simulink model "EB_12B"  (R2021b)
settings: Solver=ode3  StartTime=0.0  StopTime=0  FixedStep=.01  RelTol=1e-3  EnableMultiTasking=on
model workspace (MAT data in the model file):
  I = [1  0  0; 0  1  0; 0  0  1]
  I0 = [0  0  0; 0  0  0; 0  0  0]
  N = 18
  Wp = [1  0  0  0  0; 0  1  0  0  0; 0  0  1  0  0; 0  0  0  1  0; 0  0  0  0  1]
  X = [-0.000916135593528 0.000741784354662 -0.000111198836647 -0.000114918934981 -0.000338802758293 0.00087934621238 0.000425682524619 0.000877814042518 6.19118807071e-05 -0.000956394036441 0.000640782162368 -0.000425007884451 0.000734759332255 0.000720421624474 0.000101264737043]
  cmd.Wp = [1  0  0  0  0; 0  1  0  0  0; 0  0  1  0  0; 0  0  0  1  0; 0  0  0  0  1]
  cmd.d = [3; -1; 2]
  cmd.up = [0; 0; 0; 0; 0]
  cmd.I0 = [0  0  0; 0  0  0; 0  0  0]
  cmd.I = [1  0  0; 0  1  0; 0  0  1]
  cmd.tout = 0
  cs : handle (value not decoded)
  curPath = '/Users/khouloud.gaaloul/Documents/Projects/QRA-LocalSearch/Local Search Algorithms/Problems'
  d = 16
  hws = [3707764736; 2; 1; 1; 1; 1]
  i = 7
  j = 5
  list(1).name = 'I'
  list(1).size = [3 3]
  list(1).bytes = 72
  list(1).class = 'double'
  list(1).global = 0
  list(1).sparse = 0
  list(1).complex = 0
  list(1).nesting.function = ''
  list(1).nesting.level = 1
  list(1).persistent = 0
  list(2).name = 'I0'
  list(2).size = [3 3]
  list(2).bytes = 72
  list(2).class = 'double'
  list(2).global = 0
  list(2).sparse = 0
  list(2).complex = 0
  list(2).nesting.function = ''
  list(2).nesting.level = 1
  list(2).persistent = 0
  list(3).name = 'N'
  list(3).size = [1 1]
  list(3).bytes = 8
  list(3).class = 'double'
  list(3).global = 0
  list(3).sparse = 0
  list(3).complex = 0
  list(3).nesting.function = ''
  list(3).nesting.level = 1
  list(3).persistent = 0
  list(4).name = 'Wp'
  list(4).size = [5 5]
  list(4).bytes = 200
  list(4).class = 'double'
  list(4).global = 0
  list(4).sparse = 0
  list(4).complex = 0
  list(4).nesting.function = ''
  list(4).nesting.level = 1
  list(4).persistent = 0
  list(5).name = 'cs'
  list(5).size = [1 1]
  list(5).bytes = 0
  list(5).class = 'Simulink.ConfigSet'
  list(5).global = 0
  list(5).sparse = 0
  list(5).complex = 0
  list(5).nesting.function = ''
  list(5).nesting.level = 1
  list(5).persistent = 0
  list(6).name = 'curPath'
  list(6).size = [1 91]
  list(6).bytes = 182
  list(6).class = 'char'
  list(6).global = 0
  list(6).sparse = 0
  list(6).complex = 0
  list(6).nesting.function = ''
  list(6).nesting.level = 1
  list(6).persistent = 0
  list(7).name = 'd'
  list(7).size = [3 1]
  list(7).bytes = 24
  list(7).class = 'double'
  list(7).global = 0
  list(7).sparse = 0
  list(7).complex = 0
  list(7).nesting.function = ''
  list(7).nesting.level = 1
  list(7).persistent = 0
  list(8).name = 'hws'
  list(8).size = [1 1]
  list(8).bytes = 8
  list(8).class = 'Simulink.ModelWorkspace'
  list(8).global = 0
  list(8).sparse = 0
  list(8).complex = 0
  list(8).nesting.function = ''
  list(8).nesting.level = 1
  list(8).persistent = 0
  list(9).name = 'i'
  list(9).size = [1 1]
  list(9).bytes = 8
  list(9).class = 'double'
  list(9).global = 0
  list(9).sparse = 0
  list(9).complex = 0
  list(9).nesting.function = ''
  list(9).nesting.level = 1
  list(9).persistent = 0
  list(10).name = 'j'
  list(10).size = [1 1]
  list(10).bytes = 8
  list(10).class = 'double'
  list(10).global = 0
  list(10).sparse = 0
  list(10).complex = 0
  list(10).nesting.function = ''
  list(10).nesting.level = 1
  list(10).persistent = 0
  list(11).name = 'list'
  list(11).size = [18 1]
  list(11).bytes = 26158
  list(11).class = 'struct'
  list(11).global = 0
  list(11).sparse = 0
  list(11).complex = 0
  list(11).nesting.function = ''
  list(11).nesting.level = 1
  list(11).persistent = 0
  list(12).name = 'model_cs'
  list(12).size = [1 1]
  list(12).bytes = 0
  list(12).class = 'Simulink.ConfigSet'
  list(12).global = 0
  list(12).sparse = 0
  list(12).complex = 0
  list(12).nesting.function = ''
  list(12).nesting.level = 1
  list(12).persistent = 0
  list(13).name = 'modelpath'
  list(13).size = [1 80]
  list(13).bytes = 160
  list(13).class = 'char'
  list(13).global = 0
  list(13).sparse = 0
  list(13).complex = 0
  list(13).nesting.function = ''
  list(13).nesting.level = 1
  list(13).persistent = 0
  list(14).name = 'simOut'
  list(14).size = [1 1]
  list(14).bytes = 10925
  list(14).class = 'Simulink.SimulationOutput'
  list(14).global = 0
  list(14).sparse = 0
  list(14).complex = 0
  list(14).nesting.function = ''
  list(14).nesting.level = 1
  list(14).persistent = 0
  list(15).name = 'tout'
  list(15).size = [1 1]
  list(15).bytes = 8
  list(15).class = 'double'
  list(15).global = 0
  list(15).sparse = 0
  list(15).complex = 0
  list(15).nesting.function = ''
  list(15).nesting.level = 1
  list(15).persistent = 0
  list(16).name = 'up'
  list(16).size = [5 1]
  list(16).bytes = 40
  list(16).class = 'double'
  list(16).global = 0
  list(16).sparse = 0
  list(16).complex = 0
  list(16).nesting.function = ''
  list(16).nesting.level = 1
  list(16).persistent = 0
  list(17).name = 'var'
  list(17).size = [3 5]
  list(17).bytes = 120
  list(17).class = 'double'
  list(17).global = 0
  list(17).sparse = 0
  list(17).complex = 0
  list(17).nesting.function = ''
  list(17).nesting.level = 1
  list(17).persistent = 0
  list(18).name = 'varout'
  list(18).size = [1 1]
  list(18).bytes = 4323
  list(18).class = 'struct'
  list(18).global = 0
  list(18).sparse = 0
  list(18).complex = 0
  list(18).nesting.function = ''
  list(18).nesting.level = 1
  list(18).persistent = 0
  model_cs : handle (value not decoded)
  modelpath = '/Users/khouloud.gaaloul/Documents/Projects/QRA-LocalSearch/Simulink Models/6_eb/'
  req = 'R2'
  simOut = Simulink.SimulationOutput
  simOut.Data.tout = 0
  simOut.Data.varout.time = 0
  simOut.Data.varout.signals(1).values = [0  0  0; 0  0  0; 0  0  0]
  simOut.Data.varout.signals(1).dimensions = [3 3]
  simOut.Data.varout.signals(1).label = ''
  simOut.Data.varout.signals(1).blockName = 'EB_12B/check'
  simOut.Data.varout.signals(2).values = [1000000000000  0  0; 0  1000000000000  0; 0  0  1000000000000]
  simOut.Data.varout.signals(2).dimensions = [3 3]
  simOut.Data.varout.signals(2).label = ''
  simOut.Data.varout.signals(2).blockName = 'EB_12B/yinv'
  simOut.Data.varout.signals(3).values = [0  0  0; 0  0  0; 0  0  0; 0  0  0; 0  0  0]
  simOut.Data.varout.signals(3).dimensions = [5 3]
  simOut.Data.varout.signals(3).label = ''
  simOut.Data.varout.signals(3).blockName = 'EB_12B/P'
  simOut.Data.varout.signals(4).values = [0 0 0 0 0]
  simOut.Data.varout.signals(4).dimensions = 5
  simOut.Data.varout.signals(4).label = ''
  simOut.Data.varout.signals(4).blockName = 'EB_12B/u'
  simOut.Data.varout.signals(5).values = [-3 1 -2]
  simOut.Data.varout.signals(5).dimensions = 3
  simOut.Data.varout.signals(5).label = ''
  simOut.Data.varout.signals(5).blockName = 'EB_12B/Buminusd'
  simOut.Data.varout.signals(6).values = 0
  simOut.Data.varout.signals(6).dimensions = 1
  simOut.Data.varout.signals(6).label = ''
  simOut.Data.varout.signals(6).blockName = 'EB_12B/J'
  simOut.Data.varout.signals(7).values = 1
  simOut.Data.varout.signals(7).dimensions = 1
  simOut.Data.varout.signals(7).label = ''
  simOut.Data.varout.signals(7).blockName = 'EB_12B/ridge_on'
  simOut.Metadata = Simulink.SimulationMetadata
  simOut.Metadata.ModelInfo.ModelName = 'EB_12B'
  simOut.Metadata.ModelInfo.ModelVersion = '1.70'
  simOut.Metadata.ModelInfo.ModelFilePath = '/Users/khouloud.gaaloul/Documents/Projects/QRA-LocalSearch/Simulink Models/6_eb/EB_12B.slx'
  simOut.Metadata.ModelInfo.UserID = 'khouloud.gaaloul'
  simOut.Metadata.ModelInfo.MachineName = ''
  simOut.Metadata.ModelInfo.Platform = 'MACI64'
  simOut.Metadata.ModelInfo.ModelStructuralChecksum = [893138603; 2259620877; 265752267; 1923685794]
  simOut.Metadata.ModelInfo.SimulationMode = 'normal'
  simOut.Metadata.ModelInfo.StartTime = 0
  simOut.Metadata.ModelInfo.StopTime = 0
  simOut.Metadata.ModelInfo.SolverInfo.Type = 'Fixed-Step'
  simOut.Metadata.ModelInfo.SolverInfo.Solver = 'FixedStepDiscrete'
  simOut.Metadata.ModelInfo.SolverInfo.FixedStepSize = 0.01
  simOut.Metadata.ModelInfo.SimulinkVersion.Name = 'Simulink'
  simOut.Metadata.ModelInfo.SimulinkVersion.Version = '9.1'
  simOut.Metadata.ModelInfo.SimulinkVersion.Release = '(R2018a)'
  simOut.Metadata.ModelInfo.SimulinkVersion.Date = '06-Feb-2018'
  simOut.Metadata.ModelInfo.LoggingInfo.LoggingToFile = 'off'
  simOut.Metadata.TimingInfo.WallClockTimestampStart = '2018-11-07 17:57:54.082518'
  simOut.Metadata.TimingInfo.WallClockTimestampStop = '2018-11-07 17:57:54.533264'
  simOut.Metadata.TimingInfo.InitializationElapsedWallTime = 0.383556
  simOut.Metadata.TimingInfo.ExecutionElapsedWallTime = 0.000319
  simOut.Metadata.TimingInfo.TerminationElapsedWallTime = 0.066881
  simOut.Metadata.TimingInfo.TotalElapsedWallTime = 0.450756
  simOut.Metadata.ExecutionInfo.StopEvent = 'ReachedStopTime'
  simOut.Metadata.ExecutionInfo.StopEventSource = []
  simOut.Metadata.ExecutionInfo.StopEventDescription = 'Reached stop time of 0'
  simOut.Metadata.ExecutionInfo.ErrorDiagnostic = []
  simOut.Metadata.ExecutionInfo.WarningDiagnostics = struct([])
  simOut.Metadata.AppInfo = struct()
  tout = 0
  up = [0; 0; 0; 0; 0]
  var.time = 0
  var.signals.values = [-0.000916135593528  0.000741784354662  -0.000111198836647  -0.000114918934981  -0.000338802758293; 0.00087934621238  0.000425682524619  0.000877814042518  6.19118807071e-05  -0.000956394036441; 0.000640782162368  -0.000425007884451  0.000734759332255  0.000720421624474  0.000101264737043]
  var.signals.dimensions = [3 5]
  varout.time = 0
  varout.signals(1).values = [0  0  0; 0  0  0; 0  0  0]
  varout.signals(1).dimensions = [3 3]
  varout.signals(1).label = ''
  varout.signals(1).blockName = 'EB_12B/check'
  varout.signals(2).values = [1000000000000  0  0; 0  1000000000000  0; 0  0  1000000000000]
  varout.signals(2).dimensions = [3 3]
  varout.signals(2).label = ''
  varout.signals(2).blockName = 'EB_12B/yinv'
  varout.signals(3).values = [0  0  0; 0  0  0; 0  0  0; 0  0  0; 0  0  0]
  varout.signals(3).dimensions = [5 3]
  varout.signals(3).label = ''
  varout.signals(3).blockName = 'EB_12B/P'
  varout.signals(4).values = [0 0 0 0 0]
  varout.signals(4).dimensions = 5
  varout.signals(4).label = ''
  varout.signals(4).blockName = 'EB_12B/u'
  varout.signals(5).values = [-3 1 -2]
  varout.signals(5).dimensions = 3
  varout.signals(5).label = ''
  varout.signals(5).blockName = 'EB_12B/Buminusd'
  varout.signals(6).values = 0
  varout.signals(6).dimensions = 1
  varout.signals(6).label = ''
  varout.signals(6).blockName = 'EB_12B/J'
  varout.signals(7).values = 1
  varout.signals(7).dimensions = 1
  varout.signals(7).label = ''
  varout.signals(7).blockName = 'EB_12B/ridge_on'
  vars = {'Wp'; 'd'; 'up'; 'I0'; 'I'; 'tout'}
settings Model: Creator=elliocm  LastModifiedBy=yangy
settings SolverCC: AlgebraicLoopSolver=TrustRegion
settings DataIOCC: ExternalInput=aoe_tsinghua_mhi_data  LimitDataPoints=on  LoadExternalInput=on  SaveFormat=StructureWithTime  SignalLoggingSaveFormat=ModelDataLogs  ReturnWorkspaceOutputs=off
settings OptimizationCC: LifeSpan=inf
settings DebuggingCC: UnderspecifiedInitializationDetection=Classic  MergeDetectMultiDrivingBlocksExec=none  SolverPrmCheckMsg=warning  MultiTaskDSMMsg=warning  MultiTaskCondExecSysMsg=none  SFUnexpectedBacktrackingDiag=warning  SFNoUnconditionalDefaultTransitionDiag=warning  SFExecutionAtInitializationDiag=none  SFMachineParentedDataDiag=warning  ArithmeticOperatorsInVariantConditions=warning
settings HardwareCC: ProdBitPerPointer=32  ProdBitPerSizeT=32  ProdBitPerPtrDiffT=32  ProdLargestAtomicFloat=None  ProdIntDivRoundTo=Undefined  ProdEndianess=Unspecified  ProdWordSize=32  ProdHWDeviceType=32-bit Generic
settings ModelReferenceCC: PropagateSignalLabelsOutOfModel=off
settings SFSimCC: SimUseLocalCustomCode=off  CustomCodeUndefinedFunction=UseInterfaceOnly
settings RTWCC: RTWUseLocalCustomCode=off
settings CodeAppCC: StateflowObjectComments=on
settings GRTTargetCC: TargetLangStandard=C89/C90 (ANSI)
settings ConfigComp: CovMetricSettings=dw  CovSaveCumulativeToWorkspaceVar=on  CovSaveSingleToWorkspaceVar=on  CovExternalEMLEnable=off

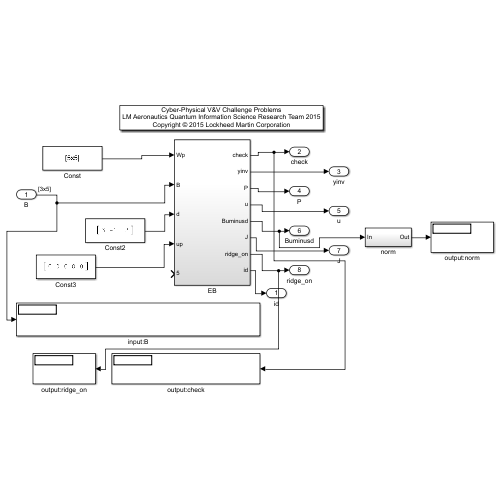
[thumbnail: Simulink's stored preview of the top-level diagram]
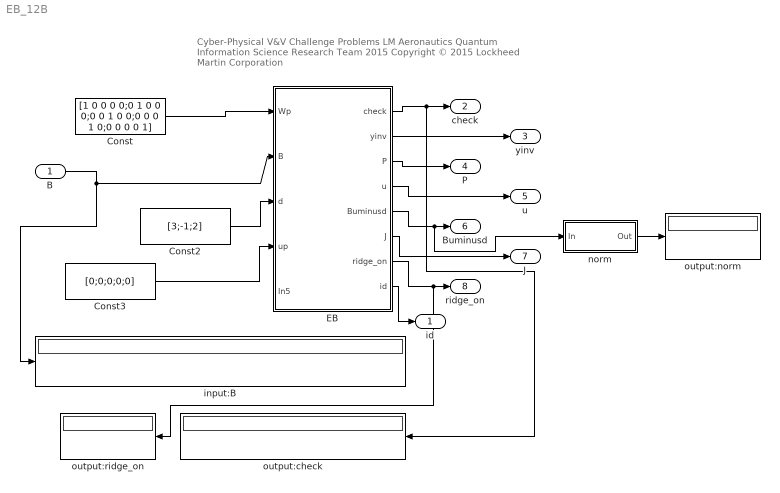
== system EB_12B ==
  note: Cyber-Physical V&V Challenge Problems
      | LM Aeronautics Quantum Information Science Research Team 2015
      | Copyright © 2015 Lockheed Martin Corporation
  B : Inport  OutDataTypeStr=double  PortDimensions=[3 5]
  Const : Constant  Value=[1 0 0 0 0;0 1 0 0 0;0 0 1 0 0;0 0 0 1 0;0 0 0 0 1]
  Const2 : Constant  Value=[3;-1;2]
  Const3 : Constant  Value=[0;0;0;0;0]
  EB : Subsystem
  input:B : Display
      settings: Decimation=6
  norm : Subsystem
  output:check : Display
      settings: Decimation=6
  output:norm : Display
      settings: Decimation=6
  output:ridge_on : Display
      settings: Decimation=6
  id : Outport  VectorParamsAs1DForOutWhenUnconnected=off
  check : Outport  Port=2  VectorParamsAs1DForOutWhenUnconnected=off
  yinv : Outport  Port=3  VectorParamsAs1DForOutWhenUnconnected=off
  P : Outport  Port=4  VectorParamsAs1DForOutWhenUnconnected=off
  u : Outport  Port=5  VectorParamsAs1DForOutWhenUnconnected=off
  Buminusd : Outport  Port=6  VectorParamsAs1DForOutWhenUnconnected=off
  J : Outport  Port=7  VectorParamsAs1DForOutWhenUnconnected=off
  ridge_on : Outport  Port=8  VectorParamsAs1DForOutWhenUnconnected=off
  wires:
  Const/1 -> EB/1(Wp)
  B/1 -> input:B/1, EB/2(B)
  EB/2(yinv) -> yinv/1
  EB/1(check) -> output:check/1, check/1
  Const2/1 -> EB/3(d)
  EB/3(P) -> P/1
  EB/4(u) -> u/1
  Const3/1 -> EB/4(up)
  EB/5(Buminusd) -> norm/1(In), Buminusd/1
  EB/6(J) -> J/1
  EB/7(ridge_on) -> output:ridge_on/1, ridge_on/1
  norm/1(Out) -> output:norm/1
  EB/8(id) -> id/1

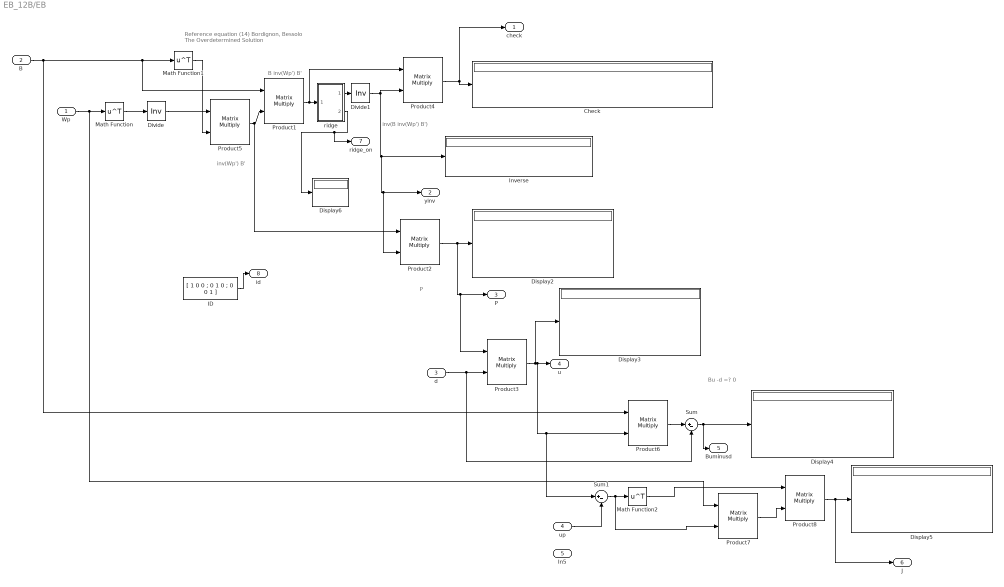
== system EB_12B/EB ==
  note: Reference equation (14) Bordignon, Bessolo
      | The Overdetermined Solution
  note: Bu -d =? 0
  note: P
  note: B inv(Wp') B'
  note: inv(B inv(Wp') B')
  note: inv(Wp') B'
  Wp : Inport
  B : Inport  Port=2
  d : Inport  Port=3
  up : Inport  Port=4
  In5 : Inport  Port=5
  Check : Display
      settings: Decimation=15
  Display{2..6} (5 alike) : Display
  Divide : Product  Inputs=/  Multiplication=Matrix(*)
  Divide1 : Product  Inputs=/  Multiplication=Matrix(*)
  ID : Constant  Value=[ 1 0 0 ; 0 1 0 ; 0 0 1 ]
  Inverse : Display
  Math Function : Math  Operator=transpose  SignedPower=on  SaturateOnIntegerOverflow=on
  Math Function1 : Math  Operator=transpose  SignedPower=on  SaturateOnIntegerOverflow=on
  Math Function2 : Math  Operator=transpose  SignedPower=on  SaturateOnIntegerOverflow=on
  Product{1..8} (8 alike) : Product  Multiplication=Matrix(*)
  Sum : Sum  Inputs=|+-
  Sum1 : Sum  Inputs=|+-
  ridge : Subsystem
  check : Outport  VectorParamsAs1DForOutWhenUnconnected=off
  yinv : Outport  Port=2  VectorParamsAs1DForOutWhenUnconnected=off
  P : Outport  Port=3  VectorParamsAs1DForOutWhenUnconnected=off
  u : Outport  Port=4  VectorParamsAs1DForOutWhenUnconnected=off
  Buminusd : Outport  Port=5  VectorParamsAs1DForOutWhenUnconnected=off
  J : Outport  Port=6  VectorParamsAs1DForOutWhenUnconnected=off
  ridge_on : Outport  Port=7  VectorParamsAs1DForOutWhenUnconnected=off
  id : Outport  Port=8  VectorParamsAs1DForOutWhenUnconnected=off
  wires:
  Product1/1 -> Product4/1, ridge/1(In1)
  ridge/1(Out1) -> Divide1/1
  Divide/1 -> Product5/1
  Divide1/1 -> Product2/2, yinv/1, Inverse/1, Product4/2
  Math Function1/1 -> Product5/2
  B/1 -> Product6/1, Product1/1, Math Function1/1
  Math Function/1 -> Divide/1
  Wp/1 -> Product7/1, Math Function/1
  Product5/1 -> Product2/1, Product1/2
  Product4/1 -> check/1, Check/1
  Product2/1 -> Product3/1, P/1, Display2/1
  d/1 -> Sum/2, Product3/2
  Product3/1 -> Display3/1, Sum1/1, Product6/2, u/1
  Product6/1 -> Sum/1
  Sum/1 -> Buminusd/1, Display4/1
  up/1 -> Sum1/2
  Sum1/1 -> Product7/2, Math Function2/1
  Math Function2/1 -> Product8/1
  Product7/1 -> Product8/2
  Product8/1 -> J/1, Display5/1
  ridge/2(ridge_on) -> ridge_on/1, Display6/1
  ID/1 -> id/1

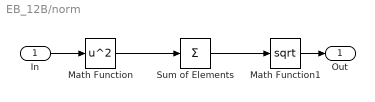
== system EB_12B/norm ==
  In : Inport
  Math Function : Math  Operator=square  SignedPower=on  SaturateOnIntegerOverflow=on
  Math Function1 : Math  Operator=sqrt  SignedPower=on  SaturateOnIntegerOverflow=on
  Sum of Elements : Sum  Inputs=+
  Out : Outport  VectorParamsAs1DForOutWhenUnconnected=off
  wires:
  Math Function/1 -> Sum of Elements/1
  Sum of Elements/1 -> Math Function1/1
  In/1 -> Math Function/1
  Math Function1/1 -> Out/1

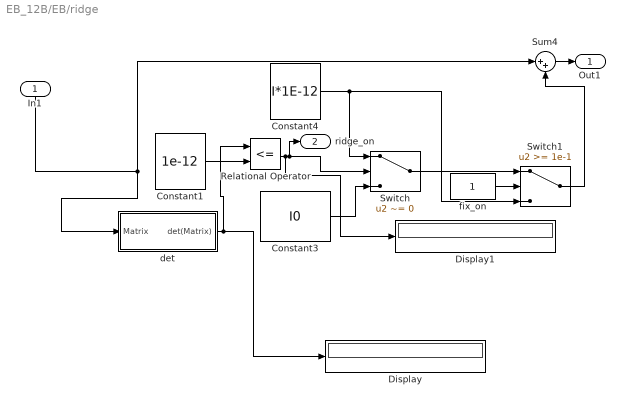
== system EB_12B/EB/ridge ==
  In1 : Inport
  Constant1 : Constant  Value=1e-12
  Constant3 : Constant  Value=I0
  Constant4 : Constant  Value=I*1E-12
  Display : Display
  Display1 : Display
  Relational Operator : RelationalOperator  Operator=<=  OutDataTypeStr=boolean  RndMeth=Nearest
  Sum4 : Sum  Inputs=|++
  Switch : Switch  Criteria=u2 ~= 0  Threshold=1e-5
  Switch1 : Switch  Threshold=1e-1
  det : Subsystem
  fix_on : Constant
  Out1 : Outport  VectorParamsAs1DForOutWhenUnconnected=off
  ridge_on : Outport  Port=2  VectorParamsAs1DForOutWhenUnconnected=off
  wires:
  Sum4/1 -> Out1/1
  Constant4/1 -> Switch/1, Switch1/3
  In1/1 -> Sum4/1, det/1(Matrix)
  Switch1/1 -> Sum4/2
  Switch/1 -> Switch1/1
  fix_on/1 -> Switch1/2
  det/1(det(Matrix)) -> Relational Operator/1, Display/1
  Relational Operator/1 -> Display1/1, ridge_on/1, Switch/2
  Constant1/1 -> Relational Operator/2
  Constant3/1 -> Switch/3

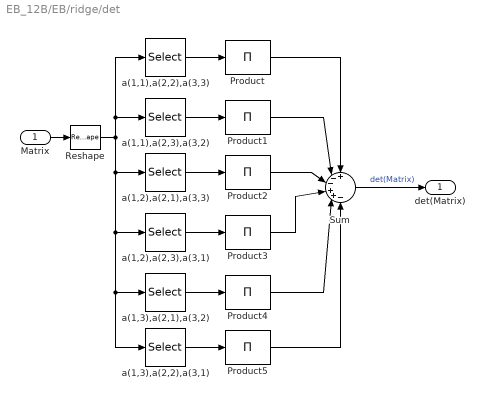
== system EB_12B/EB/ridge/det ==
  Matrix : Inport  PortDimensions=[3 3]
  Product{,1..5} (6 alike) : Product  Inputs=1  SaturateOnIntegerOverflow=on  OutDataTypeStr=Inherit: Same as first input
  Reshape : Reshape  OutputDimensionality=Column vector (2-D)
  Sum : Sum  Inputs=+--++-  SaturateOnIntegerOverflow=on
  a(1,1),a(2,2),a(3,3) : Selector  InputPortWidth=9  IndexOptions=Index vector (dialog)  Indices=[1 5 9]  OutputSizes=1
  a(1,1),a(2,3),a(3,2) : Selector  InputPortWidth=9  IndexOptions=Index vector (dialog)  Indices=[1 6 8]  OutputSizes=1
  a(1,2),a(2,1),a(3,3) : Selector  InputPortWidth=9  IndexOptions=Index vector (dialog)  Indices=[2 4 9]  OutputSizes=1
  a(1,2),a(2,3),a(3,1) : Selector  InputPortWidth=9  IndexOptions=Index vector (dialog)  Indices=[3 4 8]  OutputSizes=1
  a(1,3),a(2,1),a(3,2) : Selector  InputPortWidth=9  IndexOptions=Index vector (dialog)  Indices=[2 6 7]  OutputSizes=1
  a(1,3),a(2,2),a(3,1) : Selector  InputPortWidth=9  IndexOptions=Index vector (dialog)  Indices=[3 5 7]  OutputSizes=1
  det(Matrix) : Outport  PortDimensions=1  VectorParamsAs1DForOutWhenUnconnected=off
  wires:
  a(1,1),a(2,2),a(3,3)/1 -> Product/1
  a(1,1),a(2,3),a(3,2)/1 -> Product1/1
  a(1,2),a(2,1),a(3,3)/1 -> Product2/1
  a(1,2),a(2,3),a(3,1)/1 -> Product3/1
  a(1,3),a(2,1),a(3,2)/1 -> Product4/1
  a(1,3),a(2,2),a(3,1)/1 -> Product5/1
  Product/1 -> Sum/1
  Product1/1 -> Sum/2
  Product2/1 -> Sum/3
  Product3/1 -> Sum/4
  Product4/1 -> Sum/5
  Product5/1 -> Sum/6
  Matrix/1 -> Reshape/1
  Sum/1 -> det(Matrix)/1  "det(Matrix)"
  Reshape/1 -> a(1,1),a(2,2),a(3,3)/1, a(1,1),a(2,3),a(3,2)/1, a(1,2),a(2,1),a(3,3)/1, a(1,2),a(2,3),a(3,1)/1, a(1,3),a(2,1),a(3,2)/1, a(1,3),a(2,2),a(3,1)/1
